simulink model "feedForwardControl"  (R2018a)
settings: Solver=VariableStepAuto  StartTime=0.0  StopTime=300  RelTol=1e-3
libraries: cstblocks x7
settings Model: Creator=Haydar  LastModifiedBy=Haydar

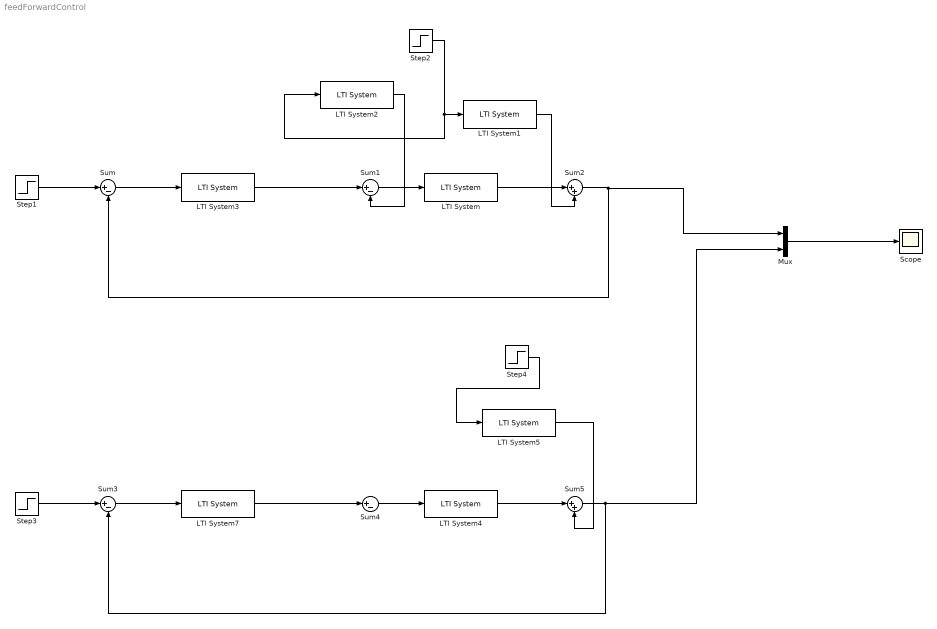
== system feedForwardControl ==
  LTI System : cstblocks/LTI System  sys=G  IC=[]
  LTI System1 : cstblocks/LTI System  sys=Gd  IC=[]
  LTI System2 : cstblocks/LTI System  sys=Gf  IC=[]
  LTI System3 : cstblocks/LTI System  sys=C  IC=[]
  LTI System4 : cstblocks/LTI System  sys=G  IC=[]
  LTI System5 : cstblocks/LTI System  sys=Gd  IC=[]
  LTI System7 : cstblocks/LTI System  sys=C  IC=[]
  Mux : Mux  Inputs=2
  Scope : Scope
  Step1 : Step  SampleTime=0
  Step2 : Step  Time=100  SampleTime=0
  Step3 : Step  SampleTime=0
  Step4 : Step  Time=100  SampleTime=0
  Sum{,1,3..4} (4 alike) : Sum  Inputs=|+-
  Sum2 : Sum  Inputs=|++
  Sum5 : Sum  Inputs=|++
  wires:
  Sum/1 -> LTI System3/1
  LTI System3/1 -> Sum1/1
  Sum1/1 -> LTI System/1
  LTI System1/1 -> Sum2/2
  Step1/1 -> Sum/1
  Step2/1 -> LTI System2/1, LTI System1/1
  LTI System2/1 -> Sum1/2
  LTI System/1 -> Sum2/1
  Sum2/1 -> Mux/1, Sum/2
  Step4/1 -> LTI System5/1
  Step3/1 -> Sum3/1
  LTI System5/1 -> Sum5/2
  LTI System4/1 -> Sum5/1
  LTI System7/1 -> Sum4/1
  Sum3/1 -> LTI System7/1
  Sum4/1 -> LTI System4/1
  Sum5/1 -> Mux/2, Sum3/2
  Mux/1 -> Scope/1
